simulink model "ex4_p202"  (R2020b)
settings: Solver=VariableStepAuto  StartTime=0.0  StopTime=0.4096  RelTol=1e-3
libraries: dsparch4 x1, dspfdesign x1, dspsrcs4 x1
settings Model: Creator=seojoon  LastModifiedBy=seojoon

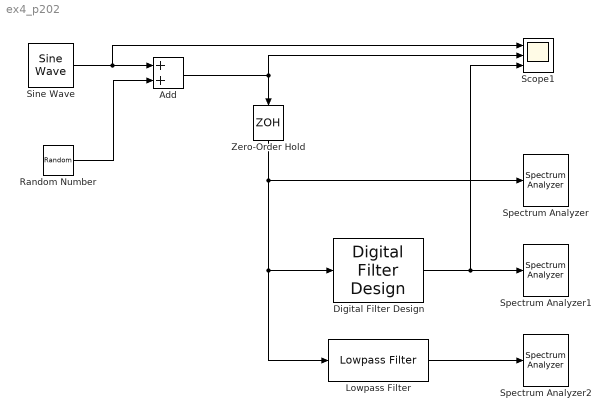
== system ex4_p202 ==
  Add : Sum
  Digital Filter Design : dsparch4/Digital Filter Design  mwdsp_browser_bugfix_var=off
  Lowpass Filter : dspfdesign/Lowpass Filter  FilterType=FIR  DesignForMinimumOrder=on  FilterOrder=50  PassbandFrequency=8e3  StopbandFrequency=12e3  PassbandRipple=0.1  StopbandAttenuation=80  InheritSampleRate=off  SampleRate=44100  SimulateUsing=Interpreted execution  roundingMode=Floor  coeffsDataTypeStr=fixdt(1,16)
  Random Number : RandomNumber  SampleTime=1e-5
  Scope1 : Scope  NumInputPorts=3
  Sine Wave : dspsrcs4/Sine Wave  Amplitude=10  Frequency=1000  Phase=0  SampleMode=Discrete  OutComplex=Real  CompMethod=Trigonometric fcn  TableSize=Speed  SampleTime=1/10000  SamplesPerFrame=1  ResetState=Restart at time zero  OutputFrames=off  dataType=double  wordLen=16  udDataType=sfix(16)  fracBitsMode=Best precision  numFracBits=15  OutDataTypeStr=double  LastOutDataTypeStr=double
  Spectrum Analyzer : SpectrumAnalyzer
  Spectrum Analyzer1 : SpectrumAnalyzer
  Spectrum Analyzer2 : SpectrumAnalyzer
  Zero-Order Hold : ZeroOrderHold  SampleTime=1e-4
  wires:
  Sine Wave/1 -> Scope1/1, Add/1
  Random Number/1 -> Add/2
  Add/1 -> Scope1/2, Zero-Order Hold/1
  Zero-Order Hold/1 -> Spectrum Analyzer/1, Lowpass Filter/1, Digital Filter Design/1
  Digital Filter Design/1 -> Scope1/3, Spectrum Analyzer1/1
  Lowpass Filter/1 -> Spectrum Analyzer2/1
